simulink model "calc_tau"  (R2020b)
settings: Solver=FixedStepDiscrete  StartTime=0.0  StopTime=stopTime  FixedStep=2.0833333333333333e-05  RelTol=1e-3
values from neighbouring files (symbols this model uses):
  centerfreq = 165.4*(10^((bmplace+1.2)/(35/2.1))-1.0)    [modelparameters.m]
  cf = 1000    [modelparameters.m]
  cohc = 1    [modelparameters.m]
  TauWBMax = taumin+0.2*(taumax-taumin)    [modelparameters.m]
  TauWBMin = TauWBMax/taumax*taumin    [modelparameters.m]
  tdres = 1/Fs    (= 2.08333333333e-05)    [modelparameters.m]
  TWOPI = 6.28318530717959    (= 6.28318530718)    [modelparameters.m]
undefined symbols (not defined in the file or in its folder): bmTaumax, bmTaumin, mp, wbgain_i
libraries: simulink x2, hdlsllib x2
settings Model: Creator=Ross  LastModifiedBy=tyler
settings DataIOCC: SaveOutput=off  SaveTime=off  ReturnWorkspaceOutputs=off
settings OptimizationCC: BlockReduction=off  ConditionallyExecuteInputs=off  DefaultParameterBehavior=Inlined
settings DebuggingCC: ReadBeforeWriteMsg=DisableAll  WriteAfterWriteMsg=DisableAll  WriteAfterReadMsg=DisableAll  AlgebraicLoopMsg=error  MultiTaskDSMMsg=none  SingleTaskRateTransMsg=error  PregeneratedLibrarySubsystemCodeDiagnostic=none  ArithmeticOperatorsInVariantConditions=warning
settings HardwareCC: ProdBitPerPointer=32  ProdBitPerSizeT=32  ProdBitPerPtrDiffT=32  ProdLargestAtomicFloat=None  ProdIntDivRoundTo=Undefined  ProdEndianess=Unspecified  ProdWordSize=32  ProdHWDeviceType=ASIC/FPGA->ASIC/FPGA  TargetBitPerPointer=64  TargetBitPerSizeT=64  TargetBitPerPtrDiffT=64  TargetLongLongMode=on  TargetIntDivRoundTo=Zero  TargetEndianess=LittleEndian  TargetWordSize=64  TargetHWDeviceType=Custom Processor->MATLAB Host Computer  ProdEqTarget=off
settings ModelReferenceCC: UpdateModelReferenceTargets=IfOutOfDate  ModelReferenceNumInstancesAllowed=Single
settings SFSimCC: SFSimEcho=off  SimUseLocalCustomCode=off  CustomCodeUndefinedFunction=UseInterfaceOnly
settings RTWCC: RTWUseLocalCustomCode=off

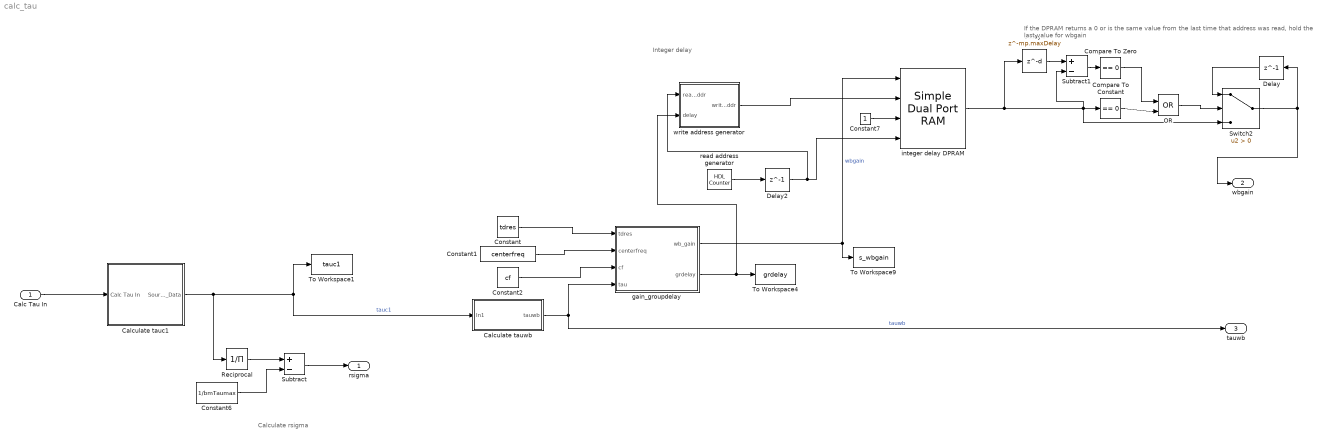
== system calc_tau ==
  note: Calculate rsigma
  note: If the DPRAM returns a 0 or is the same value from the last time that address was read, hold the last value for wbgain
  note: Integer delay
  Calc Tau In : Inport  OutDataTypeStr=single  PortDimensions=1  SampleTime=[2.0833333333333333e-05,0]
  Calculate tauc1 : Subsystem
  Calculate tauwb : Subsystem
  Compare To Constant : simulink/Logic and Bit Operations/Compare To Constant  relop===  const=0  OutDataTypeStr=boolean
  Compare To Zero : simulink/Logic and Bit Operations/Compare To Zero  relop===  OutDataTypeStr=boolean
  Constant : Constant  Value=tdres  OutDataTypeStr=single  SampleTime=-1
  Constant1 : Constant  Value=centerfreq  OutDataTypeStr=single  SampleTime=-1
  Constant2 : Constant  Value=cf  OutDataTypeStr=single  SampleTime=-1
  Constant6 : Constant  Value=1/bmTaumax  OutDataTypeStr=single  SampleTime=-1
  Constant7 : Constant  OutDataTypeStr=Inherit: Inherit via back propagation  SampleTime=-1
  Delay : Delay  DelayLength=1  InitialCondition=wbgain_i
  Delay1 : Delay  DelayLength=mp.maxDelay  InitialCondition=0
  Delay2 : Delay  DelayLength=1
  OR : Logic  Operator=OR  IconShape=distinctive  AllPortsSameDT=off  OutDataTypeStr=boolean
  Reciprocal : Product  Inputs=/  RndMeth=Zero  SaturateOnIntegerOverflow=on
  Subtract : Sum  Inputs=+-
  Subtract1 : Sum  Inputs=+-
  Switch2 : Switch  Criteria=u2 > Threshold
  To Workspace1 : ToWorkspace  VariableName=tauc1  SampleTime=-1
      settings: Save2DSignal=2-D array (concatenate along first dimension)
  To Workspace4 : ToWorkspace  VariableName=grdelay  SampleTime=-1
      settings: Save2DSignal=2-D array (concatenate along first dimension)
  To Workspace9 : ToWorkspace  VariableName=s_wbgain  SampleTime=-1
      settings: Save2DSignal=2-D array (concatenate along first dimension)
  gain_groupdelay : Subsystem
  integer delay DPRAM : hdlsllib/HDL RAMs/Simple Dual Port RAM  ram_size=mp.integerDelayAddrSize
      settings: SourceProductBaseCode=SL
  read address generator : hdlsllib/Sources/HDL Counter  CountType=Count limited  CountInit=0  CountStep=1  CountMax=mp.integerDelayBufferSize - 1  CountFromType=Initial value  CountFrom=0  CountResetPort=off  CountLoadPort=off  CountEnbPort=off  CountDirPort=off  CountDataType=Unsigned  CountWordLen=mp.integerDelayAddrSize  CountFracLen=0  CountSampTime=-1
  write address generator : Subsystem
  rsigma : Outport  OutDataTypeStr=single  PortDimensions=1  SampleTime=[2.0833333333333333e-05,0]  VectorParamsAs1DForOutWhenUnconnected=off
  wbgain : Outport  Port=2  OutDataTypeStr=single  PortDimensions=1  SampleTime=[2.0833333333333333e-05,0]  VectorParamsAs1DForOutWhenUnconnected=off
  tauwb : Outport  Port=3  OutDataTypeStr=single  PortDimensions=1  SampleTime=[2.0833333333333333e-05,0]  VectorParamsAs1DForOutWhenUnconnected=off
  wires:
  Calc Tau In/1 -> Calculate tauc1/1(Calc Tau In)
  Calculate tauc1/1(Source_Data) -> Reciprocal/1, Calculate tauwb/1(In1), To Workspace1/1  "tauc1"
  Constant/1 -> gain_groupdelay/1(tdres)
  Calculate tauwb/1(tauwb) -> tauwb/1, gain_groupdelay/4(tau)  "tauwb"
  Constant2/1 -> gain_groupdelay/3(cf)
  Constant1/1 -> gain_groupdelay/2(centerfreq)
  integer delay DPRAM/1 -> Delay1/1, Compare To Constant/1, Switch2/3, Subtract1/2
  Reciprocal/1 -> Subtract/1
  Constant6/1 -> Subtract/2
  Subtract/1 -> rsigma/1
  gain_groupdelay/2(grdelay) -> write address generator/2(delay), To Workspace4/1
  Constant7/1 -> integer delay DPRAM/3
  gain_groupdelay/1(wb_gain) -> integer delay DPRAM/1, To Workspace9/1  "wbgain"
  Delay/1 -> Switch2/1
  read address generator/1 -> Delay2/1
  write address generator/1(write_addr) -> integer delay DPRAM/2
  Switch2/1 -> Delay/1, wbgain/1
  Delay1/1 -> Subtract1/1
  Subtract1/1 -> Compare To Zero/1
  Compare To Constant/1 -> OR/2
  Compare To Zero/1 -> OR/1
  OR/1 -> Switch2/2
  Delay2/1 -> integer delay DPRAM/4, write address generator/1(read_addr)

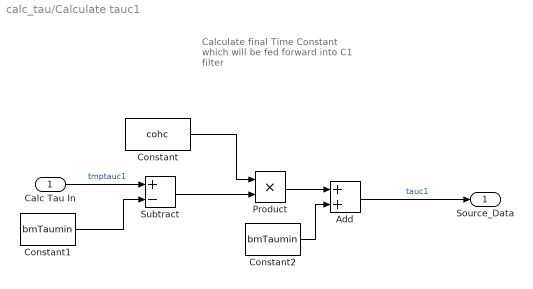
== system calc_tau/Calculate tauc1 ==
  note: Calculate final Time Constant which will be fed forward into C1 filter
  Calc Tau In : Inport
  Add : Sum
  Constant : Constant  Value=cohc  OutDataTypeStr=single  SampleTime=-1
  Constant1 : Constant  Value=bmTaumin  OutDataTypeStr=single  SampleTime=-1
  Constant2 : Constant  Value=bmTaumin  OutDataTypeStr=single  SampleTime=-1
  Product : Product
  Subtract : Sum  Inputs=+-
  Source_Data : Outport  VectorParamsAs1DForOutWhenUnconnected=off
  wires:
  Constant2/1 -> Add/2
  Subtract/1 -> Product/2
  Add/1 -> Source_Data/1  "tauc1"
  Product/1 -> Add/1
  Constant1/1 -> Subtract/2
  Constant/1 -> Product/1
  Calc Tau In/1 -> Subtract/1  "tmptauc1"

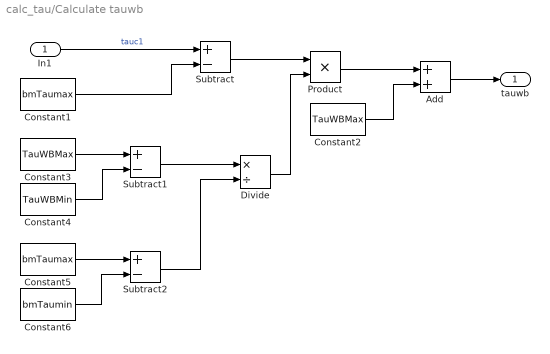
== system calc_tau/Calculate tauwb ==
  In1 : Inport
  Add : Sum
  Constant1 : Constant  Value=bmTaumax  OutDataTypeStr=single  SampleTime=-1
  Constant2 : Constant  Value=TauWBMax  OutDataTypeStr=single  SampleTime=-1
  Constant3 : Constant  Value=TauWBMax  OutDataTypeStr=single  SampleTime=-1
  Constant4 : Constant  Value=TauWBMin  OutDataTypeStr=single  SampleTime=-1
  Constant5 : Constant  Value=bmTaumax  OutDataTypeStr=single  SampleTime=-1
  Constant6 : Constant  Value=bmTaumin  OutDataTypeStr=single  SampleTime=-1
  Divide : Product  Inputs=*/  RndMeth=Zero  SaturateOnIntegerOverflow=on
  Product : Product
  Subtract : Sum  Inputs=+-
  Subtract1 : Sum  Inputs=+-
  Subtract2 : Sum  Inputs=+-
  tauwb : Outport  OutDataTypeStr=single  VectorParamsAs1DForOutWhenUnconnected=off
  wires:
  Add/1 -> tauwb/1
  Constant2/1 -> Add/2
  Divide/1 -> Product/2
  Subtract1/1 -> Divide/1
  Subtract2/1 -> Divide/2
  Constant5/1 -> Subtract2/1
  Constant6/1 -> Subtract2/2
  Constant4/1 -> Subtract1/2
  Constant3/1 -> Subtract1/1
  Subtract/1 -> Product/1
  Product/1 -> Add/1
  Constant1/1 -> Subtract/2
  In1/1 -> Subtract/1  "tauc1"

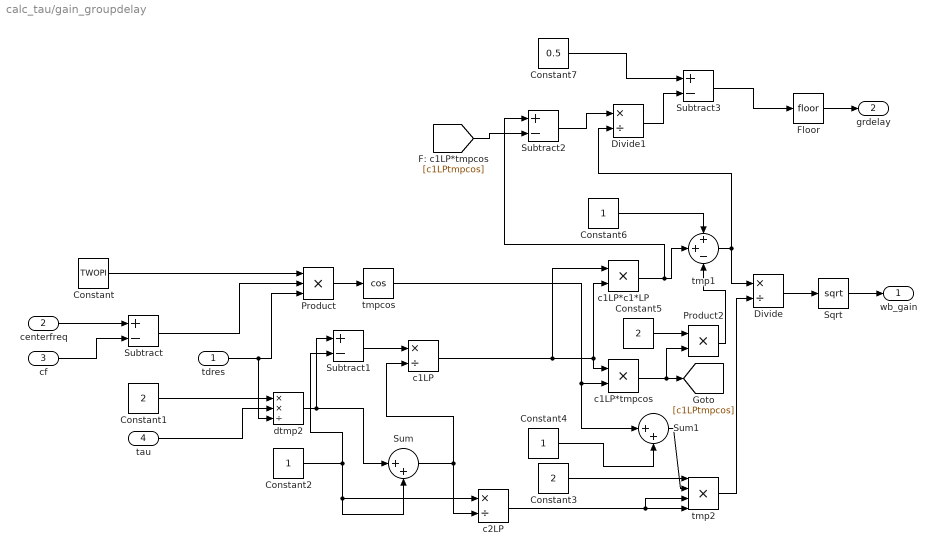
== system calc_tau/gain_groupdelay ==
  tdres : Inport
  centerfreq : Inport  Port=2
  cf : Inport  Port=3
  tau : Inport  Port=4
  Constant : Constant  Value=TWOPI  OutDataTypeStr=single  SampleTime=-1
  Constant1 : Constant  Value=2  OutDataTypeStr=single  SampleTime=-1
  Constant2 : Constant  OutDataTypeStr=single  SampleTime=-1
  Constant3 : Constant  Value=2  OutDataTypeStr=single  SampleTime=-1
  Constant4 : Constant  OutDataTypeStr=single  SampleTime=-1
  Constant5 : Constant  Value=2  OutDataTypeStr=single  SampleTime=-1
  Constant6 : Constant  OutDataTypeStr=single  SampleTime=-1
  Constant7 : Constant  Value=0.5  OutDataTypeStr=single  SampleTime=-1
  Divide : Product  Inputs=*/  RndMeth=Zero  SaturateOnIntegerOverflow=on
  Divide1 : Product  Inputs=*/  RndMeth=Zero  SaturateOnIntegerOverflow=on
  Floor : Rounding
  Product : Product  Inputs=3
  Product2 : Product
  Sqrt : Sqrt  SaturateOnIntegerOverflow=on
  Subtract{,1..3} (4 alike) : Sum  Inputs=+-
  Sum : Sum  Inputs=|++
  Sum1 : Sum  Inputs=|++
  c1LP : Product  Inputs=*/
  c1LP*c1*LP : Product
  c1LP*tmpcos : Product
  c2LP : Product  Inputs=*/  RndMeth=Zero  SaturateOnIntegerOverflow=on
  dtmp2 : Product  Inputs=**/
  tmp1 : Sum  Inputs=++-
  tmp2 : Product  Inputs=4
  tmpcos : Trigonometry  Operator=cos
  wb_gain : Outport
  grdelay : Outport  Port=2
  wires:
  Subtract3/1 -> Floor/1
  Divide1/1 -> Subtract3/2
  Subtract2/1 -> Divide1/1
  tmp1/1 -> Divide/1, Divide1/2
  Floor/1 -> grdelay/1
  Constant7/1 -> Subtract3/1
  [c1LPtmpcos] -> Subtract2/2
  Product2/1 -> tmp1/3
  Constant5/1 -> Product2/1
  Sqrt/1 -> wb_gain/1
  Divide/1 -> Sqrt/1
  tmp2/1 -> Divide/2
  Constant6/1 -> tmp1/1
  c1LP*c1*LP/1 -> tmp1/2, Subtract2/1
  c1LP*tmpcos/1 -> Product2/2, [c1LPtmpcos]
  c1LP/1 -> c1LP*c1*LP/1, c1LP*tmpcos/1, c1LP*c1*LP/2
  Sum1/1 -> tmp2/2
  tmpcos/1 -> c1LP*tmpcos/2, Sum1/1
  Constant4/1 -> Sum1/2
  c2LP/1 -> tmp2/3, tmp2/4
  Constant3/1 -> tmp2/1
  Subtract1/1 -> c1LP/1
  Constant2/1 -> Subtract1/2, Sum/2, c2LP/1
  Sum/1 -> c1LP/2, c2LP/2
  dtmp2/1 -> Subtract1/1, Sum/1
  Constant1/1 -> dtmp2/1
  tau/1 -> dtmp2/2
  Product/1 -> tmpcos/1
  tdres/1 -> dtmp2/3, Product/3
  Subtract/1 -> Product/2
  Constant/1 -> Product/1
  cf/1 -> Subtract/2
  centerfreq/1 -> Subtract/1

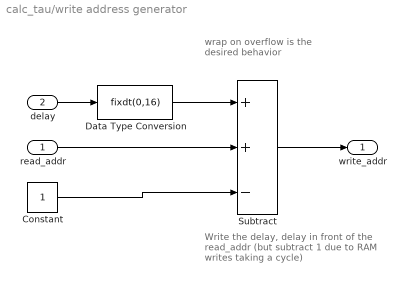
== system calc_tau/write address generator ==
  note: wrap on overflow is the desired behavior
  note: Write the delay, delay in front of the read_addr (but subtract 1 due to RAM writes taking a cycle)
  read_addr : Inport
  delay : Inport  Port=2
  Constant : Constant  OutDataTypeStr=uint16  SampleTime=-1
  Data Type Conversion : DataTypeConversion  OutMin=0  OutMax=1024  OutDataTypeStr=fixdt(0,16)  RndMeth=Nearest
  Subtract : Sum  Inputs=++-  OutDataTypeStr=Inherit: Inherit via back propagation
  write_addr : Outport  VectorParamsAs1DForOutWhenUnconnected=off
  wires:
  Constant/1 -> Subtract/3
  Data Type Conversion/1 -> Subtract/1
  Subtract/1 -> write_addr/1
  read_addr/1 -> Subtract/2
  delay/1 -> Data Type Conversion/1
